simulink model "testerdoESU"  (R2022b)
settings: Solver=ode15s  StartTime=0.0  StopTime=10  RelTol=1e-3
values from neighbouring files (symbols this model uses):
  matrixA = table2array(matrixA(:,2:10))    [dane.m]    (also in tester23.m; wykresownik33.m; wykresownik35.m; wykresownik36.m)
settings Model: Creator=48519  LastModifiedBy=48519
settings ModelReferenceCC: EnableRefExpFcnMdlSchedulingChecks=on

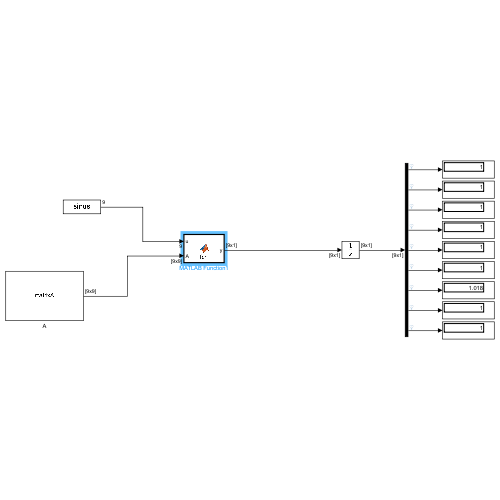
[thumbnail: Simulink's stored preview of the top-level diagram]
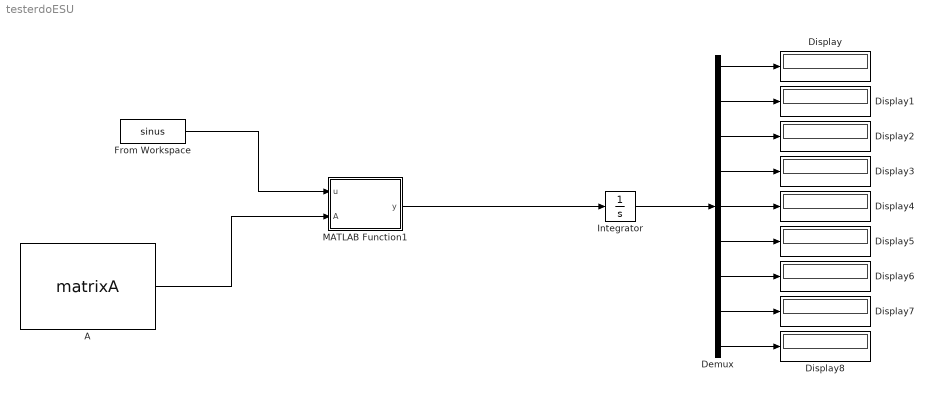
== system testerdoESU ==
  A : Constant  Value=matrixA
  Demux : Demux  Outputs=9
  Display{,1..8} (9 alike) : Display
  From Workspace : FromWorkspace  VariableName=sinus  SampleTime=0.001
  Integrator : Integrator  InitialCondition=1
  MATLAB Function1 : MATLAB Function  TreatAsAtomicUnit=on
  wires:
  A/1 -> MATLAB Function1/2(A)
  MATLAB Function1/1(y) -> Integrator/1
  Demux/5 -> Display4/1
  Demux/8 -> Display7/1
  Demux/2 -> Display1/1
  Demux/3 -> Display2/1
  Demux/6 -> Display5/1
  Demux/4 -> Display3/1
  Demux/1 -> Display/1
  Demux/9 -> Display8/1
  Integrator/1 -> Demux/1
  Demux/7 -> Display6/1
  From Workspace/1 -> MATLAB Function1/1(u)

== matlab function testerdoESU/MATLAB Function1 ==
  data: u input; y output; A input
function y = fcn(u,A)
starter=max(abs(u));
maxer=starter;
[x]=find(abs(u)==maxer,1,"first");
k= x(1,1);
i=0;
while (maxer>0.25) && (i<100)
    u=u+A*u;
    u=u+A*u;
    maxer= abs((abs(u(k))-starter))/(starter+0.1);
    i=i+1;
end
    y=u;
